simulink model "simul"  (Simulink 7.7)
settings: Solver=ode45  StartTime=0.0  StopTime=10.0  RelTol=1e-3
undefined symbols (not defined in the file): br, cr, Jr, kr
settings Model: Creator=Felipe  LastModifiedBy=Felipe

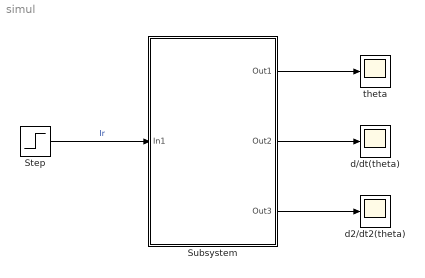
== system simul ==
  Step : Step  SampleTime=0
  Subsystem : Subsystem
  d/dt(theta) : Scope
  d2/dt2(theta) : Scope
      settings: SaveName=ScopeData2
  theta : Scope
  wires:
  Step/1 -> Subsystem/1(In1)  "Ir"
  Subsystem/1(Out1) -> theta/1
  Subsystem/2(Out2) -> d/dt(theta)/1
  Subsystem/3(Out3) -> d2/dt2(theta)/1

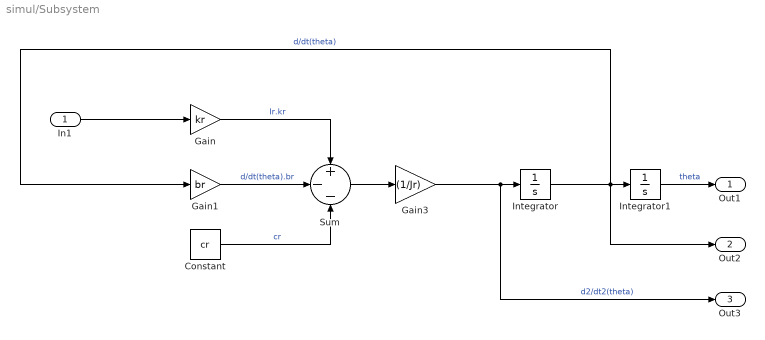
== system simul/Subsystem ==
  In1 : Inport
  Constant : Constant  Value=cr
  Gain : Gain  Gain=kr
  Gain1 : Gain  Gain=br
  Gain3 : Gain  Gain=(1/Jr)
  Integrator : Integrator
  Integrator1 : Integrator
  Sum : Sum  Inputs=+--
  Out1 : Outport
  Out2 : Outport  Port=2
  Out3 : Outport  Port=3
  wires:
  In1/1 -> Gain/1
  Gain/1 -> Sum/1  "Ir.kr"
  Gain1/1 -> Sum/2  "d/dt(theta).br"
  Constant/1 -> Sum/3  "cr"
  Sum/1 -> Gain3/1
  Gain3/1 -> Integrator/1, Out3/1  "d2/dt2(theta)"
  Integrator/1 -> Integrator1/1, Gain1/1, Out2/1  "d/dt(theta)"
  Integrator1/1 -> Out1/1  "theta"
